simulink model "Sottomarino"  (R2024b)
settings: Solver=VariableStepAuto  StartTime=0.0  StopTime=10.0  RelTol=1e-3
values from neighbouring files (symbols this model uses):
  b = 0.25    [ScriptProgetto.m]
  g = 9.81    [ScriptProgetto.m]
  K = 0.5    [ScriptProgetto.m]
  M = 3059100    [ScriptProgetto.m]
  rhoa = 1000    [ScriptProgetto.m]
  v = 9270    [ScriptProgetto.m]
  x1eq = heq    (= 0)    [ScriptProgetto.m]
  x2eq = 0    [ScriptProgetto.m]
  x3eq = meq    (= 6210900)    [ScriptProgetto.m]
settings Model: Creator=angel  LastModifiedBy=martinhaugen
settings SolverCC: AlgebraicLoopSolver=TrustRegion
settings DataIOCC: ReturnWorkspaceOutputs=off
settings DebuggingCC: UnconnectedInputMsg=warning  UnconnectedOutputMsg=warning  UnconnectedLineMsg=warning  ArithmeticOperatorsInVariantConditions=warning
settings ModelReferenceCC: EnableRefExpFcnMdlSchedulingChecks=on
settings SFSimCC: SimUseLocalCustomCode=off  CustomCodeUndefinedFunction=UseInterfaceOnly
settings RTWCC: RTWUseLocalCustomCode=off  GPUComputeCapability=3.5
settings CodeAppCC: StateflowObjectComments=on

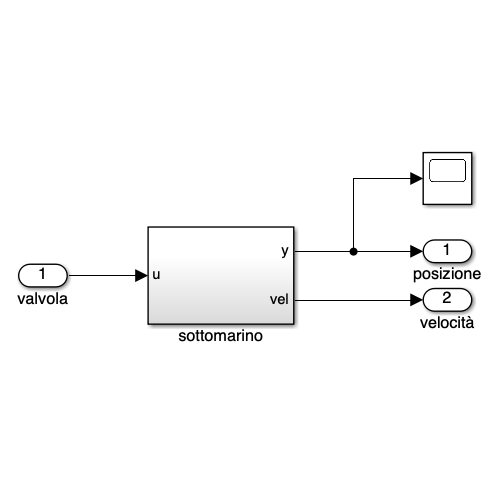
[thumbnail: Simulink's stored preview of the top-level diagram]
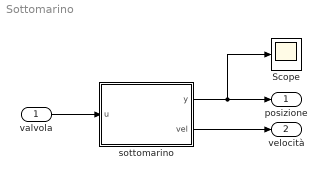
== system Sottomarino ==
  valvola : Inport
  Scope : Scope
  sottomarino : Subsystem
  posizione : Outport
  velocità : Outport  Port=2
  wires:
  valvola/1 -> sottomarino/1(u)
  sottomarino/1(y) -> Scope/1, posizione/1
  sottomarino/2(vel) -> velocità/1

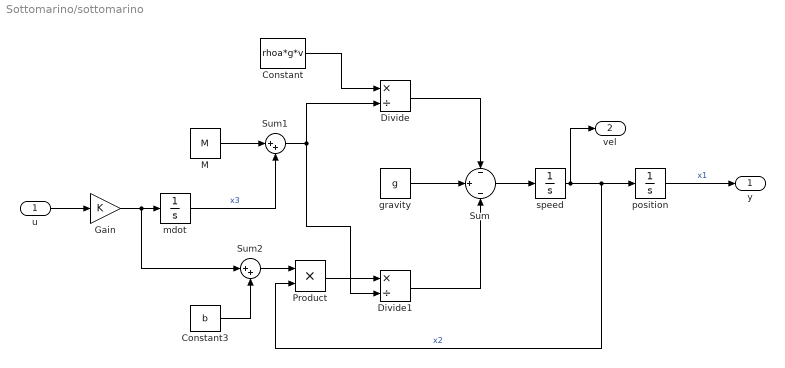
== system Sottomarino/sottomarino ==
  u : Inport
  Constant : Constant  Value=rhoa*g*v
  Constant3 : Constant  Value=b
  Divide : Product  Inputs=*/
  Divide1 : Product  Inputs=*/
  Gain : Gain  Gain=K
  M : Constant  Value=M
  Product : Product
  Sum : Sum  Inputs=-|+|-
  Sum1 : Sum  Inputs=|++
  Sum2 : Sum  Inputs=|++
  gravity : Constant  Value=g
  mdot : Integrator  InitialCondition=x3eq +100
  position : Integrator  InitialCondition=x1eq
  speed : Integrator  InitialCondition=x2eq
  y : Outport
  vel : Outport  Port=2
  wires:
  mdot/1 -> Sum1/2  "x3"
  Sum1/1 -> Divide/2, Divide1/2
  gravity/1 -> Sum/2
  Constant/1 -> Divide/1
  position/1 -> y/1  "x1"
  M/1 -> Sum1/1
  Sum2/1 -> Product/1
  u/1 -> Gain/1
  Product/1 -> Divide1/1
  speed/1 -> vel/1, position/1, Product/2  "x2"
  Divide/1 -> Sum/1
  Constant3/1 -> Sum2/2
  Sum/1 -> speed/1
  Gain/1 -> Sum2/1, mdot/1
  Divide1/1 -> Sum/3
